simulink model "Grid_PBFORCAPF_ab_Detail_2013b_616"  (R2021b)
settings: Solver=FixedStepDiscrete  StartTime=0.0  StopTime=1.5  FixedStep=Ts_Power  RelTol=1e-3
InitFcn:
  | %% Sys Para
  | N=200;fg=50;Vbase=200;
  | Ts_Control=1/N/fg;
  | Tscon=Ts_Control;
  | Ts_Power=Ts_Control/128;
  | fsw=1/Ts_Control;
  | Vdcref=350;
  | Vdcini=Vdcref;
  | 
  | 
  | 
  | %% Load Side
  | Ll=2.0e-3;Rl=1e-2;
  | RL=100;
  | 
  | %% DG Circuit Parameters
  | %% LCL
  | L1_DG1=1.4e-3;R1=1e-3;
  | L2_DG1=0.4e-3;R2=1e-3;
  | Cx_DG1=6.3e-6;
  | 
  | L1_DG2=L1_DG1;L2_DG2=L2_DG1;Cx_DG2=Cx_DG1;
  | L1_DG3=L1_DG1;L2_DG3=L2_DG1;Cx_DG3=Cx_DG1;
  | Cdc=0.55e-3;
  | %PLL;
  | Kp_pll=88;
  | Ki_pll=0.4/Ts_Control;
  | 
  | %% DG2 Controller Parameters
  | Kpc_DG1=4.89;
  | Kic_DG1=0;
  | 
  | Kpdc_DG1=0.2;
  | Kidc_DG1=0.1;
undefined symbols (not defined in the file or in its folder): DiscIntNeverNeededParam, L2, Rd
libraries: spsThreePhaseSeriesRLCBranchLib x13, slpidlib x8, spsThreePhaseVIMeasurementLib x8, spsStairGeneratorLib x8, simulink x6, simulink_extras x6, spsSeriesRLCBranchLib x5, spsThreePhaseBreakerLib x5, spsUniversalBridgeLib x4, spsNeutralLib x4, spsGroundLib x3, spsPWMGenerator2LevelLib x3
(part 3 of 3)

== system Grid_PBFORCAPF_ab_Detail_2013b_616/Controller1/SV Modulator Pattern #1/Determine the sector of U* based on alpha (rad). Also, determine if the sector number is odd ==
  alpha : Inport
  Constant1 : Constant  Value=2
  Look-Up Table : Lookup  InputValues=[0:pi/3:5*pi/3]  Table=[1:6]  SaturateOnIntegerOverflow=on
  Math Function1 : Math  Operator=mod  SignedPower=on  SaturateOnIntegerOverflow=on
  Rounding Function : Rounding
  Sn : Outport  VectorParamsAs1DForOutWhenUnconnected=off
  Odd_S : Outport  Port=2  VectorParamsAs1DForOutWhenUnconnected=off
  wires:
  alpha/1 -> Look-Up Table/1
  Math Function1/1 -> Odd_S/1
  Constant1/1 -> Math Function1/2
  Rounding Function/1 -> Sn/1, Math Function1/1
  Look-Up Table/1 -> Rounding Function/1

== system Grid_PBFORCAPF_ab_Detail_2013b_616/Controller1/SV Modulator Pattern #1/Generate pulse pattern ==
  note: D1
  note: D2
  note: D0D0D0
  Sn : Inport
  D120 : Inport  Port=2
  Demux1 : Demux  Outputs=3
      settings: DisplayOption=none
  Multiport Switch : MultiPortSwitch  Inputs=6  SaturateOnIntegerOverflow=on  InputSameDT=on
  Multiport Switch1 : MultiPortSwitch  Inputs=6  SaturateOnIntegerOverflow=on  InputSameDT=on
  Multiport Switch2 : MultiPortSwitch  Inputs=6  SaturateOnIntegerOverflow=on  InputSameDT=on
  Mux1 : Mux  Inputs=3
  abc : Outport  VectorParamsAs1DForOutWhenUnconnected=off
  wires:
  D120/1 -> Demux1/1
  Sn/1 -> Multiport Switch1/1, Multiport Switch2/1, Multiport Switch/1
  Multiport Switch/1 -> Mux1/1
  Multiport Switch2/1 -> Mux1/3
  Multiport Switch1/1 -> Mux1/2
  Demux1/1 -> Multiport Switch/7, Multiport Switch1/3, Multiport Switch1/4, Multiport Switch2/6, Multiport Switch2/5, Multiport Switch/2
  Demux1/2 -> Multiport Switch/3, Multiport Switch/6, Multiport Switch1/2, Multiport Switch1/5, Multiport Switch2/4, Multiport Switch2/7
  Demux1/3 -> Multiport Switch/4, Multiport Switch/5, Multiport Switch1/6, Multiport Switch1/7, Multiport Switch2/3, Multiport Switch2/2
  Mux1/1 -> abc/1

== system Grid_PBFORCAPF_ab_Detail_2013b_616/Controller1/SV Modulator Pattern #1/INFO ==
  note: Interval 7
  note: Interval 6
  note: Interval 5
  note: Interval 4
  note: Interval 3
  note: Interval 2
  note: Interval 1
  note: zero
      | space vector
      | (Q1 Q3 Q5 =0)
  note: 1st basic
      | space vector
  note: 2nd basic
      | space vector
  note: zero
      | space vector
      | (Q1 Q3 Q5 =1)
  note: zero
      | space vector
      | (Q1 Q3 Q5 =0)
  note: 2nd basic
      | space vector
  note: 1st basic
      | space vector
  note: Pattern #1 implements the following symmetrical switching pattern:
      | total duration = 1 PWM period (Tpwm = 1/Fc)
  note: |
      | |
      | |
      | |
      | |
      | |
      | |
      | |
      | |
      | |
  note: |
      | |
      | |
      | |
      | |
      | |
      | |
      | |
      | |
      | |
  note: |
      | |
      | |
      | |
      | |
      | |
      | |
      | |
      | |
      | |
  note: |
      | |
      | |
      | |
      | |
      | |
      | |
      | |
      | |
      | |
  note: |
      | |
      | |
      | |
      | |
      | |
      | |
      | |
      | |
      | |
  note: |
      | |
      | |
      | |
      | |
      | |
      | |
      | |
      | |
      | |
  note: Ta/2
  note: To/4
  note: Tb/2
  note: To/2
  note: Tb/2
  note: Ta/2
  note: To/4
  note: Ta=m*cos(alpha+30)* (1/Fc)
  note: Tb=m*sin(alpha) * (1/Fc)
  note: To=(1/Fc-Ta-Tb)
  note: where:
      | Fc = Chopping frequency
      | m = modulation index
      | alpha = angle between reference vector U* and
      | 1st basic space vector

== system Grid_PBFORCAPF_ab_Detail_2013b_616/Controller1/SV Modulator Pattern #1/Subsystem ==
  TaTbTo : Inport
  " 1/2" : Gain  Gain=0.5  SaturateOnIntegerOverflow=on  OutDataTypeStr=Inherit: Same as input  ParamDataTypeStr=Inherit: Same as input
  Demux : Demux  Outputs=3
      settings: DisplayOption=none
  Mux1 : Mux  Inputs=3
  Sum5 : Sum  SaturateOnIntegerOverflow=on
  Sum6 : Sum  SaturateOnIntegerOverflow=on
  D1D2D0 : Outport  VectorParamsAs1DForOutWhenUnconnected=off
  wires:
  Demux/3 -> " 1/2"/1
  TaTbTo/1 -> Demux/1
  Sum5/1 -> Mux1/1
  Mux1/1 -> D1D2D0/1
  " 1/2"/1 -> Sum6/2, Mux1/3
  Sum6/1 -> Sum5/2, Mux1/2
  Demux/1 -> Sum5/1
  Demux/2 -> Sum6/1

== system Grid_PBFORCAPF_ab_Detail_2013b_616/Controller2/DSOGI/QSOGI ==
  v : Inport
  2 : Gain  Gain=2
  2*pi*h*Ts : Gain  Gain=6.28*h*Ts
  Constant : Constant  SampleTime=Tscon
  Constant1 : Constant  Value=50  SampleTime=Tscon
  Discrete-Time Integrator : DiscreteIntegrator  IntegratorMethod=Accumulation: Backward Euler  SampleTime=-1  ICPrevOutput=DiscIntNeverNeededParam  ICPrevScaledInput=DiscIntNeverNeededParam
  Discrete-Time Integrator1 : DiscreteIntegrator  IntegratorMethod=Accumulation: Forward Euler  SampleTime=-1  ICPrevOutput=DiscIntNeverNeededParam  ICPrevScaledInput=DiscIntNeverNeededParam
  KIh : Gain  Gain=KIh*Ts
  Product1 : Product
  Sum1 : Sum  Inputs=|+-
  Sum2 : Sum  Inputs=|+-
  Sum3 : Sum  Inputs=-+|
  Sum4 : Sum  Inputs=|++
  Sum5 : Sum  Inputs=|++
  cos(314*h*Ts)-1 : Gain  Gain=cos(314*h*Ts)-1
  cos(314*h*Ts+phch)-cos(phch) : Gain  Gain=cos(314*h*Ts+phch)-cos(phch)
  cos(phch) : Gain  Gain=cos(phch)
  cos(wh*Ts) : Trigonometry  Operator=cos
  wc : Gain  Gain=wc
  vh : Outport  VectorParamsAs1DForOutWhenUnconnected=off
  wires:
  cos(314*h*Ts)-1/1 -> Sum5/1
  Sum5/1 -> wc/1
  Sum3/1 -> KIh/1
  wc/1 -> Sum3/1
  Sum4/1 -> vh/1
  cos(314*h*Ts+phch)-cos(phch)/1 -> Sum4/2
  cos(phch)/1 -> Sum4/1
  2/1 -> Product1/1
  Sum1/1 -> 2/1
  Constant/1 -> Sum1/1
  cos(wh*Ts)/1 -> Sum1/2
  2*pi*h*Ts/1 -> cos(wh*Ts)/1
  Discrete-Time Integrator/1 -> Product1/2, cos(314*h*Ts+phch)-cos(phch)/1, cos(314*h*Ts)-1/1
  Discrete-Time Integrator1/1 -> Sum5/2, cos(phch)/1, Discrete-Time Integrator/1
  Constant1/1 -> 2*pi*h*Ts/1
  KIh/1 -> Sum2/1
  v/1 -> Sum3/2
  Sum2/1 -> Discrete-Time Integrator1/1
  Product1/1 -> Sum2/2

== system Grid_PBFORCAPF_ab_Detail_2013b_616/Controller2/FORCAB/Seperated1 ==
  fi : Inport
  Compare To Constant : simulink/Logic and Bit Operations/Compare To Constant  relop=>=  const=50  OutDataTypeStr=boolean
  Compare To Constant1 : simulink/Logic and Bit Operations/Compare To Constant  relop=<  const=-10  OutDataTypeStr=boolean
  Constant : Constant  Value=1/Ts_Control  SampleTime=Tscon
  Data Type Conversion : DataTypeConversion  OutDataTypeStr=double
  Data Type Conversion1 : DataTypeConversion  OutDataTypeStr=double
  Discrete-Time Integrator : DiscreteIntegrator  gainval=1/Ts_Control  ExternalReset=level  InitialCondition=200  SampleTime=-1  LimitOutput=on  UpperSaturationLimit=300  LowerSaturationLimit=100  ICPrevOutput=DiscIntNeverNeededParam  ICPrevScaledInput=DiscIntNeverNeededParam
  N=1/f0/Ts : Fcn  Expr=1/u(1)/Ts
  Product2 : Product
  Sum3 : Sum  Inputs=+-
  Sum4 : Sum  Inputs=+-
  Ni : Outport  VectorParamsAs1DForOutWhenUnconnected=off
  N : Outport  Port=2  VectorParamsAs1DForOutWhenUnconnected=off
  wires:
  Data Type Conversion/1 -> Sum4/1
  Discrete-Time Integrator/1 -> Product2/2, Ni/1  "Ni2"
  [RSTT2] -> Discrete-Time Integrator/2
  Compare To Constant/1 -> Data Type Conversion/1
  Sum3/1 -> Compare To Constant1/1, Compare To Constant/1
  fi/1 -> Product2/1, N=1/f0/Ts/1
  Compare To Constant1/1 -> Data Type Conversion1/1
  Data Type Conversion1/1 -> Sum4/2
  Sum4/1 -> Discrete-Time Integrator/1
  N=1/f0/Ts/1 -> N/1
  Constant/1 -> Sum3/1
  Product2/1 -> Sum3/2

== system Grid_PBFORCAPF_ab_Detail_2013b_616/Controller2/FORCAB/Subsystem1 ==
  In : Inport
  F : Inport  Port=2
  1-F : Fcn  Expr=1-u(1)
  Product : Product
  Product1 : Product
  Sum3 : Sum
  Unit Delay1 : UnitDelay  SampleTime=-1  HasFrameUpgradeWarning=on
  Out : Outport  VectorParamsAs1DForOutWhenUnconnected=off
  wires:
  Product1/1 -> Sum3/2
  Unit Delay1/1 -> Product/1
  Sum3/1 -> Out/1
  1-F/1 -> Product1/2
  In/1 -> Unit Delay1/1, Product1/1
  Product/1 -> Sum3/1
  F/1 -> Product/2, 1-F/1

== system Grid_PBFORCAPF_ab_Detail_2013b_616/Controller2/SV Modulator Pattern #1/Compute time duration of switching states (Ta,Tb,To)  ==
  note: Ta=m*cos(alpha+30)* (1/Fc)
  note: Tb=m*sin(alpha) * (1/Fc)
  note: To=(1/Fc-Ta-Tb)
  note: TaTbTo
  alpha : Inport
  m : Inport  Port=2
  Sn : Inport  Port=3
  Odd_S : Inport  Port=4
  Constant : Constant  Value=pi/6
  Constant1 : Constant  Value=pi/3
  Constant2 : Constant
  Constant8 : Constant
  Mux : Mux  Inputs=2
  Mux1 : Mux  Inputs=2
  Product : Product  SaturateOnIntegerOverflow=on  OutDataTypeStr=Inherit: Same as first input
  Product1 : Product  SaturateOnIntegerOverflow=on  OutDataTypeStr=Inherit: Same as first input
  Selector1 : Selector  InputPortWidth=3  IndexOptions=Index vector (dialog)  Indices=[2 1 3]  OutputSizes=1
  Sum : Sum  SaturateOnIntegerOverflow=on
  Sum1 : Sum  Inputs=+-  SaturateOnIntegerOverflow=on
  Sum2 : Sum  Inputs=1  SaturateOnIntegerOverflow=on
  Sum3 : Sum  Inputs=-+  SaturateOnIntegerOverflow=on
  Sum4 : Sum  Inputs=+-  SaturateOnIntegerOverflow=on
  Switch1 : Switch  Threshold=0.5  SaturateOnIntegerOverflow=on
  Trigonometric Function : Trigonometry
  Trigonometric Function1 : Trigonometry  Operator=cos
  Ta_Tb_To : Outport  VectorParamsAs1DForOutWhenUnconnected=off
  tag scope: alpha2=global
  wires:
  Trigonometric Function1/1 -> Mux/1
  Trigonometric Function/1 -> Mux/2
  Mux/1 -> Product/2
  m/1 -> Product/1
  Sum/1 -> Trigonometric Function1/1
  Sum2/1 -> Sum3/1
  Constant8/1 -> Sum3/2
  Sum1/1 -> Product1/1
  Constant1/1 -> Product1/2
  Sn/1 -> Sum1/1
  Constant2/1 -> Sum1/2
  Product1/1 -> Sum4/2
  alpha/1 -> Sum4/1
  Product/1 -> Mux1/1, Sum2/1  "TaTb"
  Sum3/1 -> Mux1/2  "To"
  Sum4/1 -> Sum/1, Trigonometric Function/1, [alpha2]  "alpha"
  Constant/1 -> Sum/2
  Mux1/1 -> Switch1/1, Selector1/1
  Selector1/1 -> Switch1/3
  Switch1/1 -> Ta_Tb_To/1
  Odd_S/1 -> Switch1/2

== system Grid_PBFORCAPF_ab_Detail_2013b_616/Controller2/SV Modulator Pattern #1/Determine the sector of U* based on alpha (rad). Also, determine if the sector number is odd ==
  alpha : Inport
  Constant1 : Constant  Value=2
  Look-Up Table : Lookup  InputValues=[0:pi/3:5*pi/3]  Table=[1:6]  SaturateOnIntegerOverflow=on
  Math Function1 : Math  Operator=mod  SignedPower=on  SaturateOnIntegerOverflow=on
  Rounding Function : Rounding
  Sn : Outport  VectorParamsAs1DForOutWhenUnconnected=off
  Odd_S : Outport  Port=2  VectorParamsAs1DForOutWhenUnconnected=off
  wires:
  Look-Up Table/1 -> Rounding Function/1
  Rounding Function/1 -> Math Function1/1, Sn/1
  Constant1/1 -> Math Function1/2
  Math Function1/1 -> Odd_S/1
  alpha/1 -> Look-Up Table/1

== system Grid_PBFORCAPF_ab_Detail_2013b_616/Controller2/SV Modulator Pattern #1/Generate pulse pattern ==
  note: D0D0D0
  note: D2
  note: D1
  Sn : Inport
  D120 : Inport  Port=2
  Demux1 : Demux  Outputs=3
      settings: DisplayOption=none
  Multiport Switch : MultiPortSwitch  Inputs=6  SaturateOnIntegerOverflow=on  InputSameDT=on
  Multiport Switch1 : MultiPortSwitch  Inputs=6  SaturateOnIntegerOverflow=on  InputSameDT=on
  Multiport Switch2 : MultiPortSwitch  Inputs=6  SaturateOnIntegerOverflow=on  InputSameDT=on
  Mux1 : Mux  Inputs=3
  abc : Outport  VectorParamsAs1DForOutWhenUnconnected=off
  wires:
  Mux1/1 -> abc/1
  Demux1/3 -> Multiport Switch2/2, Multiport Switch2/3, Multiport Switch1/7, Multiport Switch1/6, Multiport Switch/5, Multiport Switch/4
  Demux1/2 -> Multiport Switch2/7, Multiport Switch2/4, Multiport Switch1/5, Multiport Switch1/2, Multiport Switch/6, Multiport Switch/3
  Demux1/1 -> Multiport Switch/2, Multiport Switch2/5, Multiport Switch2/6, Multiport Switch1/4, Multiport Switch1/3, Multiport Switch/7
  Multiport Switch1/1 -> Mux1/2
  Multiport Switch2/1 -> Mux1/3
  Multiport Switch/1 -> Mux1/1
  Sn/1 -> Multiport Switch/1, Multiport Switch2/1, Multiport Switch1/1
  D120/1 -> Demux1/1

== system Grid_PBFORCAPF_ab_Detail_2013b_616/Controller2/SV Modulator Pattern #1/INFO ==
  note: where:
      | Fc = Chopping frequency
      | m = modulation index
      | alpha = angle between reference vector U* and
      | 1st basic space vector
  note: To=(1/Fc-Ta-Tb)
  note: Tb=m*sin(alpha) * (1/Fc)
  note: Ta=m*cos(alpha+30)* (1/Fc)
  note: To/4
  note: Ta/2
  note: Tb/2
  note: To/2
  note: Tb/2
  note: To/4
  note: Ta/2
  note: |
      | |
      | |
      | |
      | |
      | |
      | |
      | |
      | |
      | |
  note: |
      | |
      | |
      | |
      | |
      | |
      | |
      | |
      | |
      | |
  note: |
      | |
      | |
      | |
      | |
      | |
      | |
      | |
      | |
      | |
  note: |
      | |
      | |
      | |
      | |
      | |
      | |
      | |
      | |
      | |
  note: |
      | |
      | |
      | |
      | |
      | |
      | |
      | |
      | |
      | |
  note: |
      | |
      | |
      | |
      | |
      | |
      | |
      | |
      | |
      | |
  note: Pattern #1 implements the following symmetrical switching pattern:
      | total duration = 1 PWM period (Tpwm = 1/Fc)
  note: 1st basic
      | space vector
  note: 2nd basic
      | space vector
  note: zero
      | space vector
      | (Q1 Q3 Q5 =0)
  note: zero
      | space vector
      | (Q1 Q3 Q5 =1)
  note: 2nd basic
      | space vector
  note: 1st basic
      | space vector
  note: zero
      | space vector
      | (Q1 Q3 Q5 =0)
  note: Interval 1
  note: Interval 2
  note: Interval 3
  note: Interval 4
  note: Interval 5
  note: Interval 6
  note: Interval 7

== system Grid_PBFORCAPF_ab_Detail_2013b_616/Controller2/SV Modulator Pattern #1/Subsystem ==
  TaTbTo : Inport
  " 1/2" : Gain  Gain=0.5  SaturateOnIntegerOverflow=on  OutDataTypeStr=Inherit: Same as input  ParamDataTypeStr=Inherit: Same as input
  Demux : Demux  Outputs=3
      settings: DisplayOption=none
  Mux1 : Mux  Inputs=3
  Sum5 : Sum  SaturateOnIntegerOverflow=on
  Sum6 : Sum  SaturateOnIntegerOverflow=on
  D1D2D0 : Outport  VectorParamsAs1DForOutWhenUnconnected=off
  wires:
  Demux/2 -> Sum6/1
  Demux/1 -> Sum5/1
  Sum6/1 -> Mux1/2, Sum5/2
  " 1/2"/1 -> Mux1/3, Sum6/2
  Mux1/1 -> D1D2D0/1
  Sum5/1 -> Mux1/1
  TaTbTo/1 -> Demux/1
  Demux/3 -> " 1/2"/1

== system Grid_PBFORCAPF_ab_Detail_2013b_616/Controller3/DSOGI/QSOGI ==
  v : Inport
  2 : Gain  Gain=2
  2*pi*h*Ts : Gain  Gain=6.28*h*Ts
  Constant : Constant  SampleTime=Tscon
  Constant1 : Constant  Value=50  SampleTime=Tscon
  Discrete-Time Integrator : DiscreteIntegrator  IntegratorMethod=Accumulation: Backward Euler  SampleTime=-1  ICPrevOutput=DiscIntNeverNeededParam  ICPrevScaledInput=DiscIntNeverNeededParam
  Discrete-Time Integrator1 : DiscreteIntegrator  IntegratorMethod=Accumulation: Forward Euler  SampleTime=-1  ICPrevOutput=DiscIntNeverNeededParam  ICPrevScaledInput=DiscIntNeverNeededParam
  KIh : Gain  Gain=KIh*Ts
  Product1 : Product
  Sum1 : Sum  Inputs=|+-
  Sum2 : Sum  Inputs=|+-
  Sum3 : Sum  Inputs=-+|
  Sum4 : Sum  Inputs=|++
  Sum5 : Sum  Inputs=|++
  cos(314*h*Ts)-1 : Gain  Gain=cos(314*h*Ts)-1
  cos(314*h*Ts+phch)-cos(phch) : Gain  Gain=cos(314*h*Ts+phch)-cos(phch)
  cos(phch) : Gain  Gain=cos(phch)
  cos(wh*Ts) : Trigonometry  Operator=cos
  wc : Gain  Gain=wc
  vh : Outport  VectorParamsAs1DForOutWhenUnconnected=off
  wires:
  Product1/1 -> Sum2/2
  Sum2/1 -> Discrete-Time Integrator1/1
  v/1 -> Sum3/2
  KIh/1 -> Sum2/1
  Constant1/1 -> 2*pi*h*Ts/1
  Discrete-Time Integrator1/1 -> Discrete-Time Integrator/1, cos(phch)/1, Sum5/2
  Discrete-Time Integrator/1 -> cos(314*h*Ts)-1/1, cos(314*h*Ts+phch)-cos(phch)/1, Product1/2
  2*pi*h*Ts/1 -> cos(wh*Ts)/1
  cos(wh*Ts)/1 -> Sum1/2
  Constant/1 -> Sum1/1
  Sum1/1 -> 2/1
  2/1 -> Product1/1
  cos(phch)/1 -> Sum4/1
  cos(314*h*Ts+phch)-cos(phch)/1 -> Sum4/2
  Sum4/1 -> vh/1
  wc/1 -> Sum3/1
  Sum3/1 -> KIh/1
  Sum5/1 -> wc/1
  cos(314*h*Ts)-1/1 -> Sum5/1

== system Grid_PBFORCAPF_ab_Detail_2013b_616/Controller3/FORCAB/Seperated1 ==
  fi : Inport
  Compare To Constant : simulink/Logic and Bit Operations/Compare To Constant  relop=>=  const=50  OutDataTypeStr=boolean
  Compare To Constant1 : simulink/Logic and Bit Operations/Compare To Constant  relop=<  const=-10  OutDataTypeStr=boolean
  Constant : Constant  Value=1/Ts_Control  SampleTime=Tscon
  Data Type Conversion : DataTypeConversion  OutDataTypeStr=double
  Data Type Conversion1 : DataTypeConversion  OutDataTypeStr=double
  Discrete-Time Integrator : DiscreteIntegrator  gainval=1/Ts_Control  ExternalReset=level  InitialCondition=200  SampleTime=-1  LimitOutput=on  UpperSaturationLimit=300  LowerSaturationLimit=100  ICPrevOutput=DiscIntNeverNeededParam  ICPrevScaledInput=DiscIntNeverNeededParam
  N=1/f0/Ts : Fcn  Expr=1/u(1)/Ts
  Product2 : Product
  Sum3 : Sum  Inputs=+-
  Sum4 : Sum  Inputs=+-
  Ni : Outport  VectorParamsAs1DForOutWhenUnconnected=off
  N : Outport  Port=2  VectorParamsAs1DForOutWhenUnconnected=off
  wires:
  Product2/1 -> Sum3/2
  Constant/1 -> Sum3/1
  N=1/f0/Ts/1 -> N/1
  Sum4/1 -> Discrete-Time Integrator/1
  Data Type Conversion1/1 -> Sum4/2
  Compare To Constant1/1 -> Data Type Conversion1/1
  fi/1 -> N=1/f0/Ts/1, Product2/1
  Sum3/1 -> Compare To Constant/1, Compare To Constant1/1
  Compare To Constant/1 -> Data Type Conversion/1
  [RSTT3] -> Discrete-Time Integrator/2
  Discrete-Time Integrator/1 -> Ni/1, Product2/2  "Ni2"
  Data Type Conversion/1 -> Sum4/1

== system Grid_PBFORCAPF_ab_Detail_2013b_616/Controller3/FORCAB/Subsystem1 ==
  In : Inport
  F : Inport  Port=2
  1-F : Fcn  Expr=1-u(1)
  Product : Product
  Product1 : Product
  Sum3 : Sum
  Unit Delay1 : UnitDelay  SampleTime=-1  HasFrameUpgradeWarning=on
  Out : Outport  VectorParamsAs1DForOutWhenUnconnected=off
  wires:
  F/1 -> 1-F/1, Product/2
  Product/1 -> Sum3/1
  In/1 -> Product1/1, Unit Delay1/1
  1-F/1 -> Product1/2
  Sum3/1 -> Out/1
  Unit Delay1/1 -> Product/1
  Product1/1 -> Sum3/2

== system Grid_PBFORCAPF_ab_Detail_2013b_616/Controller3/SV Modulator Pattern #1/Compute time duration of switching states (Ta,Tb,To)  ==
  note: TaTbTo
  note: To=(1/Fc-Ta-Tb)
  note: Tb=m*sin(alpha) * (1/Fc)
  note: Ta=m*cos(alpha+30)* (1/Fc)
  alpha : Inport
  m : Inport  Port=2
  Sn : Inport  Port=3
  Odd_S : Inport  Port=4
  Constant : Constant  Value=pi/6
  Constant1 : Constant  Value=pi/3
  Constant2 : Constant
  Constant8 : Constant
  Mux : Mux  Inputs=2
  Mux1 : Mux  Inputs=2
  Product : Product  SaturateOnIntegerOverflow=on  OutDataTypeStr=Inherit: Same as first input
  Product1 : Product  SaturateOnIntegerOverflow=on  OutDataTypeStr=Inherit: Same as first input
  Selector1 : Selector  InputPortWidth=3  IndexOptions=Index vector (dialog)  Indices=[2 1 3]  OutputSizes=1
  Sum : Sum  SaturateOnIntegerOverflow=on
  Sum1 : Sum  Inputs=+-  SaturateOnIntegerOverflow=on
  Sum2 : Sum  Inputs=1  SaturateOnIntegerOverflow=on
  Sum3 : Sum  Inputs=-+  SaturateOnIntegerOverflow=on
  Sum4 : Sum  Inputs=+-  SaturateOnIntegerOverflow=on
  Switch1 : Switch  Threshold=0.5  SaturateOnIntegerOverflow=on
  Trigonometric Function : Trigonometry
  Trigonometric Function1 : Trigonometry  Operator=cos
  Ta_Tb_To : Outport  VectorParamsAs1DForOutWhenUnconnected=off
  tag scope: alpha3=global
  wires:
  Odd_S/1 -> Switch1/2
  Switch1/1 -> Ta_Tb_To/1
  Selector1/1 -> Switch1/3
  Mux1/1 -> Selector1/1, Switch1/1
  Constant/1 -> Sum/2
  Sum4/1 -> [alpha3], Trigonometric Function/1, Sum/1  "alpha"
  Sum3/1 -> Mux1/2  "To"
  Product/1 -> Sum2/1, Mux1/1  "TaTb"
  alpha/1 -> Sum4/1
  Product1/1 -> Sum4/2
  Constant2/1 -> Sum1/2
  Sn/1 -> Sum1/1
  Constant1/1 -> Product1/2
  Sum1/1 -> Product1/1
  Constant8/1 -> Sum3/2
  Sum2/1 -> Sum3/1
  Sum/1 -> Trigonometric Function1/1
  m/1 -> Product/1
  Mux/1 -> Product/2
  Trigonometric Function/1 -> Mux/2
  Trigonometric Function1/1 -> Mux/1

== system Grid_PBFORCAPF_ab_Detail_2013b_616/Controller3/SV Modulator Pattern #1/Determine the sector of U* based on alpha (rad). Also, determine if the sector number is odd ==
  alpha : Inport
  Constant1 : Constant  Value=2
  Look-Up Table : Lookup  InputValues=[0:pi/3:5*pi/3]  Table=[1:6]  SaturateOnIntegerOverflow=on
  Math Function1 : Math  Operator=mod  SignedPower=on  SaturateOnIntegerOverflow=on
  Rounding Function : Rounding
  Sn : Outport  VectorParamsAs1DForOutWhenUnconnected=off
  Odd_S : Outport  Port=2  VectorParamsAs1DForOutWhenUnconnected=off
  wires:
  alpha/1 -> Look-Up Table/1
  Math Function1/1 -> Odd_S/1
  Constant1/1 -> Math Function1/2
  Rounding Function/1 -> Sn/1, Math Function1/1
  Look-Up Table/1 -> Rounding Function/1

== system Grid_PBFORCAPF_ab_Detail_2013b_616/Controller3/SV Modulator Pattern #1/Generate pulse pattern ==
  note: D1
  note: D2
  note: D0D0D0
  Sn : Inport
  D120 : Inport  Port=2
  Demux1 : Demux  Outputs=3
      settings: DisplayOption=none
  Multiport Switch : MultiPortSwitch  Inputs=6  SaturateOnIntegerOverflow=on  InputSameDT=on
  Multiport Switch1 : MultiPortSwitch  Inputs=6  SaturateOnIntegerOverflow=on  InputSameDT=on
  Multiport Switch2 : MultiPortSwitch  Inputs=6  SaturateOnIntegerOverflow=on  InputSameDT=on
  Mux1 : Mux  Inputs=3
  abc : Outport  VectorParamsAs1DForOutWhenUnconnected=off
  wires:
  D120/1 -> Demux1/1
  Sn/1 -> Multiport Switch1/1, Multiport Switch2/1, Multiport Switch/1
  Multiport Switch/1 -> Mux1/1
  Multiport Switch2/1 -> Mux1/3
  Multiport Switch1/1 -> Mux1/2
  Demux1/1 -> Multiport Switch/7, Multiport Switch1/3, Multiport Switch1/4, Multiport Switch2/6, Multiport Switch2/5, Multiport Switch/2
  Demux1/2 -> Multiport Switch/3, Multiport Switch/6, Multiport Switch1/2, Multiport Switch1/5, Multiport Switch2/4, Multiport Switch2/7
  Demux1/3 -> Multiport Switch/4, Multiport Switch/5, Multiport Switch1/6, Multiport Switch1/7, Multiport Switch2/3, Multiport Switch2/2
  Mux1/1 -> abc/1

== system Grid_PBFORCAPF_ab_Detail_2013b_616/Controller3/SV Modulator Pattern #1/INFO ==
  note: Interval 7
  note: Interval 6
  note: Interval 5
  note: Interval 4
  note: Interval 3
  note: Interval 2
  note: Interval 1
  note: zero
      | space vector
      | (Q1 Q3 Q5 =0)
  note: 1st basic
      | space vector
  note: 2nd basic
      | space vector
  note: zero
      | space vector
      | (Q1 Q3 Q5 =1)
  note: zero
      | space vector
      | (Q1 Q3 Q5 =0)
  note: 2nd basic
      | space vector
  note: 1st basic
      | space vector
  note: Pattern #1 implements the following symmetrical switching pattern:
      | total duration = 1 PWM period (Tpwm = 1/Fc)
  note: |
      | |
      | |
      | |
      | |
      | |
      | |
      | |
      | |
      | |
  note: |
      | |
      | |
      | |
      | |
      | |
      | |
      | |
      | |
      | |
  note: |
      | |
      | |
      | |
      | |
      | |
      | |
      | |
      | |
      | |
  note: |
      | |
      | |
      | |
      | |
      | |
      | |
      | |
      | |
      | |
  note: |
      | |
      | |
      | |
      | |
      | |
      | |
      | |
      | |
      | |
  note: |
      | |
      | |
      | |
      | |
      | |
      | |
      | |
      | |
      | |
  note: Ta/2
  note: To/4
  note: Tb/2
  note: To/2
  note: Tb/2
  note: Ta/2
  note: To/4
  note: Ta=m*cos(alpha+30)* (1/Fc)
  note: Tb=m*sin(alpha) * (1/Fc)
  note: To=(1/Fc-Ta-Tb)
  note: where:
      | Fc = Chopping frequency
      | m = modulation index
      | alpha = angle between reference vector U* and
      | 1st basic space vector

== system Grid_PBFORCAPF_ab_Detail_2013b_616/Controller3/SV Modulator Pattern #1/Subsystem ==
  TaTbTo : Inport
  " 1/2" : Gain  Gain=0.5  SaturateOnIntegerOverflow=on  OutDataTypeStr=Inherit: Same as input  ParamDataTypeStr=Inherit: Same as input
  Demux : Demux  Outputs=3
      settings: DisplayOption=none
  Mux1 : Mux  Inputs=3
  Sum5 : Sum  SaturateOnIntegerOverflow=on
  Sum6 : Sum  SaturateOnIntegerOverflow=on
  D1D2D0 : Outport  VectorParamsAs1DForOutWhenUnconnected=off
  wires:
  Demux/3 -> " 1/2"/1
  TaTbTo/1 -> Demux/1
  Sum5/1 -> Mux1/1
  Mux1/1 -> D1D2D0/1
  " 1/2"/1 -> Sum6/2, Mux1/3
  Sum6/1 -> Sum5/2, Mux1/2
  Demux/1 -> Sum5/1
  Demux/2 -> Sum6/1

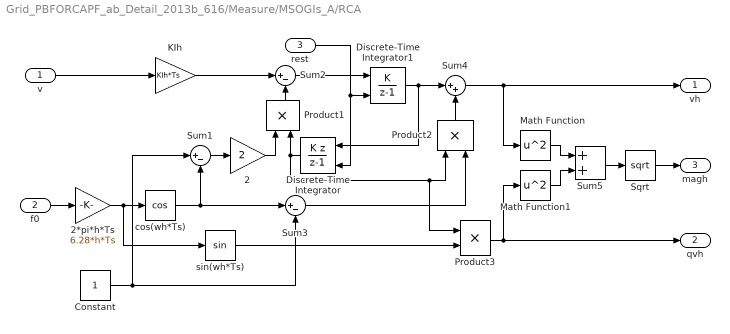
== system Grid_PBFORCAPF_ab_Detail_2013b_616/Measure/MSOGIs_A/RCA ==
  v : Inport
  f0 : Inport  Port=2
  rest : Inport  Port=3
  2 : Gain  Gain=2
  2*pi*h*Ts : Gain  Gain=6.28*h*Ts
  Constant : Constant  SampleTime=Tscon
  Discrete-Time Integrator : DiscreteIntegrator  IntegratorMethod=Accumulation: Backward Euler  ExternalReset=level  SampleTime=-1  ICPrevOutput=DiscIntNeverNeededParam  ICPrevScaledInput=DiscIntNeverNeededParam
  Discrete-Time Integrator1 : DiscreteIntegrator  IntegratorMethod=Accumulation: Forward Euler  ExternalReset=level  SampleTime=-1  ICPrevOutput=DiscIntNeverNeededParam  ICPrevScaledInput=DiscIntNeverNeededParam
  KIh : Gain  Gain=KIh*Ts
  Math Function : Math  Operator=square  SignedPower=on  SaturateOnIntegerOverflow=on
  Math Function1 : Math  Operator=square  SignedPower=on  SaturateOnIntegerOverflow=on
  Product1 : Product
  Product2 : Product
  Product3 : Product
  Sqrt : Sqrt  SaturateOnIntegerOverflow=on
  Sum1 : Sum  Inputs=|+-
  Sum2 : Sum  Inputs=|+-
  Sum3 : Sum  Inputs=|+-
  Sum4 : Sum  Inputs=|++
  Sum5 : Sum
  cos(wh*Ts) : Trigonometry  Operator=cos
  sin(wh*Ts) : Trigonometry
  vh : Outport  VectorParamsAs1DForOutWhenUnconnected=off
  qvh : Outport  Port=2  VectorParamsAs1DForOutWhenUnconnected=off
  magh : Outport  Port=3  VectorParamsAs1DForOutWhenUnconnected=off
  wires:
  rest/1 -> Discrete-Time Integrator/2, Discrete-Time Integrator1/2
  Product1/1 -> Sum2/2
  Discrete-Time Integrator/1 -> Product2/1, Product3/1, Product1/2
  Sum2/1 -> Discrete-Time Integrator1/1
  v/1 -> KIh/1
  KIh/1 -> Sum2/1
  f0/1 -> 2*pi*h*Ts/1
  Discrete-Time Integrator1/1 -> Sum4/1, Discrete-Time Integrator/1
  Product2/1 -> Sum4/2
  sin(wh*Ts)/1 -> Product3/2
  Sum4/1 -> Math Function/1, vh/1
  Product3/1 -> qvh/1, Math Function1/1
  2*pi*h*Ts/1 -> sin(wh*Ts)/1, cos(wh*Ts)/1
  cos(wh*Ts)/1 -> Sum3/1, Sum1/2
  Constant/1 -> Sum3/2, Sum1/1
  Sum1/1 -> 2/1
  2/1 -> Product1/1
  Math Function1/1 -> Sum5/2
  Math Function/1 -> Sum5/1
  Sum5/1 -> Sqrt/1
  Sqrt/1 -> magh/1
  Sum3/1 -> Product2/2

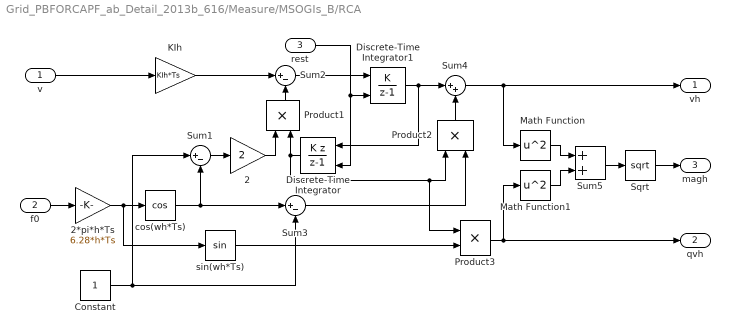
== system Grid_PBFORCAPF_ab_Detail_2013b_616/Measure/MSOGIs_B/RCA ==
  v : Inport
  f0 : Inport  Port=2
  rest : Inport  Port=3
  2 : Gain  Gain=2
  2*pi*h*Ts : Gain  Gain=6.28*h*Ts
  Constant : Constant  SampleTime=Tscon
  Discrete-Time Integrator : DiscreteIntegrator  IntegratorMethod=Accumulation: Backward Euler  ExternalReset=level  SampleTime=-1  ICPrevOutput=DiscIntNeverNeededParam  ICPrevScaledInput=DiscIntNeverNeededParam
  Discrete-Time Integrator1 : DiscreteIntegrator  IntegratorMethod=Accumulation: Forward Euler  ExternalReset=level  SampleTime=-1  ICPrevOutput=DiscIntNeverNeededParam  ICPrevScaledInput=DiscIntNeverNeededParam
  KIh : Gain  Gain=KIh*Ts
  Math Function : Math  Operator=square  SignedPower=on  SaturateOnIntegerOverflow=on
  Math Function1 : Math  Operator=square  SignedPower=on  SaturateOnIntegerOverflow=on
  Product1 : Product
  Product2 : Product
  Product3 : Product
  Sqrt : Sqrt  SaturateOnIntegerOverflow=on
  Sum1 : Sum  Inputs=|+-
  Sum2 : Sum  Inputs=|+-
  Sum3 : Sum  Inputs=|+-
  Sum4 : Sum  Inputs=|++
  Sum5 : Sum
  cos(wh*Ts) : Trigonometry  Operator=cos
  sin(wh*Ts) : Trigonometry
  vh : Outport  VectorParamsAs1DForOutWhenUnconnected=off
  qvh : Outport  Port=2  VectorParamsAs1DForOutWhenUnconnected=off
  magh : Outport  Port=3  VectorParamsAs1DForOutWhenUnconnected=off
  wires:
  Sum3/1 -> Product2/2
  Sqrt/1 -> magh/1
  Sum5/1 -> Sqrt/1
  Math Function/1 -> Sum5/1
  Math Function1/1 -> Sum5/2
  2/1 -> Product1/1
  Sum1/1 -> 2/1
  Constant/1 -> Sum1/1, Sum3/2
  cos(wh*Ts)/1 -> Sum1/2, Sum3/1
  2*pi*h*Ts/1 -> cos(wh*Ts)/1, sin(wh*Ts)/1
  Product3/1 -> Math Function1/1, qvh/1
  Sum4/1 -> vh/1, Math Function/1
  sin(wh*Ts)/1 -> Product3/2
  Product2/1 -> Sum4/2
  Discrete-Time Integrator1/1 -> Discrete-Time Integrator/1, Sum4/1
  f0/1 -> 2*pi*h*Ts/1
  KIh/1 -> Sum2/1
  v/1 -> KIh/1
  Sum2/1 -> Discrete-Time Integrator1/1
  Discrete-Time Integrator/1 -> Product1/2, Product3/1, Product2/1
  Product1/1 -> Sum2/2
  rest/1 -> Discrete-Time Integrator1/2, Discrete-Time Integrator/2
